simulink model "TractionControl"  (Simulink 8.5)
settings: Solver=ode1  StartTime=0.0  StopTime=10.0  RelTol=1e-3
libraries: simulink x1
settings Model: Creator=gwilli10  LastModifiedBy=jonah.caplan  CovSFcnEnable=off
settings DataIOCC: SignalLoggingSaveFormat=Dataset
settings OptimizationCC: BooleanDataType=off  ExpressionDepthLimit=128  OptimizeModelRefInitCode=on  LifeSpan=1
settings DebuggingCC: UnderspecifiedInitializationDetection=Simplified  MergeDetectMultiDrivingBlocksExec=error  SolverPrmCheckMsg=warning  FcnCallInpInsideContextMsg=EnableAllAsError  StateNameClashWarn=none
settings HardwareCC: ProdHWDeviceType=ASIC/FPGA->ASIC/FPGA  TargetIntDivRoundTo=Floor  TargetEndianess=LittleEndian  TargetHWDeviceType=Generic->32-bit Embedded Processor  ProdEqTarget=off
settings RTWCC: SystemTargetFile=ert.tlc  GenCodeOnly=on  TemplateMakefile=ert_default_tmf  Description=Embedded Coder  RetainRTWFile=on
settings CodeAppCC: IgnoreCustomStorageClasses=off  MATLABSourceComments=on
settings ERTTargetCC: MultiwordLength=2048  GenerateSampleERTMain=on  MultiInstanceERTCode=on  CodeInterfacePackaging=Reusable function  RootIOFormat=Structure reference  ERTCustomFileTemplate=example_file_process.tlc  ERTFilePackagingFormat=CompactWithDataFile  ConvertIfToSwitch=off  SuppressUnreachableDefaultCases=off

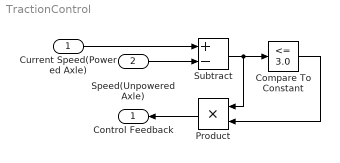
== system TractionControl ==
  Current Speed(Powered Axle) : Inport
  Speed(Unpowered Axle) : Inport  Port=2
  Compare To Constant : simulink/Logic and Bit Operations/Compare To Constant  relop=<=  const=3.0  OutDataTypeStr=boolean
  Product : Product
  Subtract : Sum  Inputs=+-  OutDataTypeStr=double
  Control Feedback : Outport
  wires:
  Subtract/1 -> Product/1, Compare To Constant/1
  Compare To Constant/1 -> Product/2
  Product/1 -> Control Feedback/1
  Speed(Unpowered Axle)/1 -> Subtract/2
  Current Speed(Powered Axle)/1 -> Subtract/1
